simulink model "fft_overlap_tomori"  (R2023b)
settings: Solver=VariableStepAuto  StartTime=0.0  StopTime=inf  RelTol=1e-3
InitFcn:
  | fftparrallelout
  | load('dataram.mat')
  | s= fi(exp(-1j*2*pi.*(0:63)/64),1,16,15);
  | fixed_point = fixdt(1,27,20);
  | fixed_pointu = fixdt(0,29,20);
  | fixed = fixdt(1,22,15);
  | const = fixdt(1,18,17);
  | addConst = fixdt(1,18,16);
  | f =10.4e6;
  | f1=45e6;
  | alpha1 =5;
  | beta1 = 0.00001 ;
  | beta2 = 0.99999 ;
  | beta3 = 23;
undefined symbols (not defined in the file or in its folder): j
libraries: dspxfrm3 x11, commrflib2 x4
(part 3 of 10)

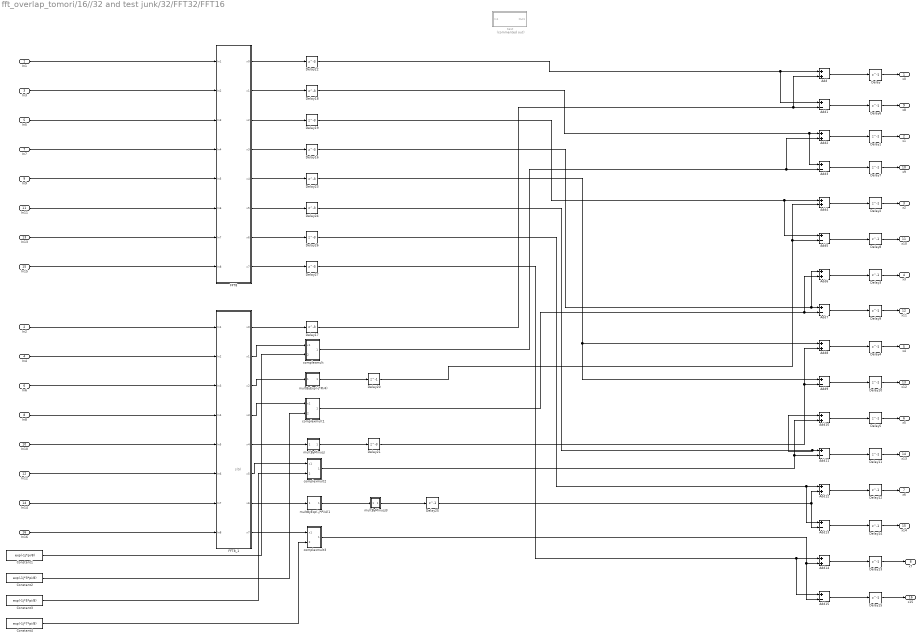
== system fft_overlap_tomori/16//32 and test junk/32/FFT32/FFT16 ==
  note: s(5)
  In1 : Inport
  In2 : Inport  Port=2
  In3 : Inport  Port=3
  In4 : Inport  Port=4
  In5 : Inport  Port=5
  In6 : Inport  Port=6
  In7 : Inport  Port=7
  In8 : Inport  Port=8
  In9 : Inport  Port=9
  In10 : Inport  Port=10
  In11 : Inport  Port=11
  In12 : Inport  Port=12
  In13 : Inport  Port=13
  In14 : Inport  Port=14
  In15 : Inport  Port=15
  In16 : Inport  Port=16
  Add{,2,4,6,8,10,12,14} (8 alike) : Sum  OutDataTypeStr=fixed
  Add{1,3,5,7,9,11,13,15} (8 alike) : Sum  Inputs=+-  OutDataTypeStr=fixed
  Constant1 : Constant  Value=exp(-1j*pi/8)  OutDataTypeStr=fixed  SampleTime=-1
  Constant2 : Constant  Value=exp(-1j*3*pi/8)  OutDataTypeStr=fixed  SampleTime=-1
  Constant3 : Constant  Value=exp(-1j*5*pi/8)  OutDataTypeStr=fixed  SampleTime=-1
  Constant4 : Constant  Value=exp(-1j*7*pi/8)  OutDataTypeStr=fixed  SampleTime=-1
  Delay{,1..15,20,25} (18 alike) : Delay  DelayLength=1
  Delay{16..19,21..24,26..27} (10 alike) : Delay  DelayLength=3
  FFT8 : Subsystem
  FFT8_1 : Subsystem
  complexmult : Subsystem
  complexmult1 : Subsystem
  complexmult2 : Subsystem
  complexmult3 : Subsystem
  multByExp(-j*Pi/4) : Subsystem
  multByExp(-j*Pi/4)1 : Subsystem
  multByMinusJ : Subsystem
  multByMinusJ3 : Subsystem
  test : Subsystem  Commented=on
  x0 : Outport
  x1 : Outport  Port=2
  x2 : Outport  Port=3
  x3 : Outport  Port=4
  x4 : Outport  Port=5
  x5 : Outport  Port=6
  x6 : Outport  Port=7
  x7 : Outport  Port=8
  x8 : Outport  Port=9
  x9 : Outport  Port=10
  x10 : Outport  Port=11
  x11 : Outport  Port=12
  x12 : Outport  Port=13
  x13 : Outport  Port=14
  x14 : Outport  Port=15
  x15 : Outport  Port=16
  wires:
  FFT8_1/1(x0) -> Delay17/1
  Add/1 -> Delay/1
  Add1/1 -> Delay6/1
  Constant1/1 -> complexmult/2(In3)
  FFT8_1/2(x1) -> complexmult/1(x1)
  FFT8/2(x1) -> Delay18/1
  Add2/1 -> Delay1/1
  complexmult/1(Out1) -> Add2/2, Add3/2
  Add3/1 -> Delay7/1
  FFT8_1/3(x2) -> multByExp(-j*Pi/4)/1(In1)
  FFT8/3(x2) -> Delay19/1
  Add4/1 -> Delay2/1
  Add5/1 -> Delay8/1
  multByExp(-j*Pi/4)/1(Out1) -> Delay20/1
  Constant2/1 -> complexmult1/2(In3)
  FFT8_1/4(x3) -> complexmult1/1(x1)
  FFT8/4(x3) -> Delay16/1
  complexmult1/1(Out1) -> Add6/2, Add7/2
  Add6/1 -> Delay3/1
  Add7/1 -> Delay9/1
  FFT8/5(x4) -> Delay23/1
  multByMinusJ/1(Out1) -> Delay21/1
  Add8/1 -> Delay4/1
  Add9/1 -> Delay10/1
  complexmult2/1(Out1) -> Add11/2, Add10/2
  FFT8/6(x5) -> Delay24/1
  Add10/1 -> Delay5/1
  Add11/1 -> Delay11/1
  Delay/1 -> x0/1
  Delay1/1 -> x1/1
  Delay2/1 -> x2/1
  Delay3/1 -> x3/1
  Delay4/1 -> x4/1
  Delay5/1 -> x5/1
  Delay6/1 -> x8/1
  Delay7/1 -> x9/1
  Delay8/1 -> x10/1
  Delay9/1 -> x11/1
  Delay10/1 -> x12/1
  Delay11/1 -> x13/1
  Delay12/1 -> x6/1
  Delay13/1 -> x7/1
  Delay14/1 -> x14/1
  Delay15/1 -> x15/1
  FFT8/1(x0) -> Delay22/1
  Delay17/1 -> Add/2, Add1/2
  Delay18/1 -> Add3/1, Add2/1
  Delay20/1 -> Add4/2, Add5/2
  Delay19/1 -> Add5/1, Add4/1
  Delay21/1 -> Add9/2, Add8/2
  FFT8_1/5(x4) -> multByMinusJ/1(x4)
  Delay22/1 -> Add1/1, Add/1
  Delay16/1 -> Add6/1, Add7/1
  Delay23/1 -> Add9/1, Add8/1
  Delay24/1 -> Add10/1, Add11/1
  FFT8_1/7(x6) -> multByExp(-j*Pi/4)1/1(In1)
  multByMinusJ3/1(Out1) -> Delay25/1
  FFT8/7(x6) -> Delay26/1
  Delay25/1 -> Add12/2, Add13/2
  Add12/1 -> Delay12/1
  Add13/1 -> Delay14/1
  Constant4/1 -> complexmult3/2(In3)
  FFT8_1/8(x7) -> complexmult3/1(x1)
  complexmult3/1(Out1) -> Add15/2, Add14/2
  FFT8/8(x7) -> Delay27/1
  Add14/1 -> Delay13/1
  Add15/1 -> Delay15/1
  Delay26/1 -> Add13/1, Add12/1
  Delay27/1 -> Add15/1, Add14/1
  FFT8_1/6(x5) -> complexmult2/1(x1)
  Constant3/1 -> complexmult2/2(In3)
  multByExp(-j*Pi/4)1/1(Out1) -> multByMinusJ3/1(In1)
  In1/1 -> FFT8/1(In1)
  In3/1 -> FFT8/2(In2)
  In5/1 -> FFT8/3(In3)
  In7/1 -> FFT8/4(In4)
  In9/1 -> FFT8/5(In5)
  In11/1 -> FFT8/6(In6)
  In13/1 -> FFT8/7(In7)
  In15/1 -> FFT8/8(In8)
  In2/1 -> FFT8_1/1(In1)
  In4/1 -> FFT8_1/2(In2)
  In6/1 -> FFT8_1/3(In3)
  In8/1 -> FFT8_1/4(In4)
  In10/1 -> FFT8_1/5(In5)
  In12/1 -> FFT8_1/6(In6)
  In14/1 -> FFT8_1/7(In7)
  In16/1 -> FFT8_1/8(In8)

== system fft_overlap_tomori/16//32 and test junk/32/FFT32/FFT16_1 ==
  note: s(5)
  In1 : Inport
  In2 : Inport  Port=2
  In3 : Inport  Port=3
  In4 : Inport  Port=4
  In5 : Inport  Port=5
  In6 : Inport  Port=6
  In7 : Inport  Port=7
  In8 : Inport  Port=8
  In9 : Inport  Port=9
  In10 : Inport  Port=10
  In11 : Inport  Port=11
  In12 : Inport  Port=12
  In13 : Inport  Port=13
  In14 : Inport  Port=14
  In15 : Inport  Port=15
  In16 : Inport  Port=16
  Add{,2,4,6,8,10,12,14} (8 alike) : Sum  OutDataTypeStr=fixed
  Add{1,3,5,7,9,11,13,15} (8 alike) : Sum  Inputs=+-  OutDataTypeStr=fixed
  Constant1 : Constant  Value=exp(-1j*pi/8)  OutDataTypeStr=fixed  SampleTime=-1
  Constant2 : Constant  Value=exp(-1j*3*pi/8)  OutDataTypeStr=fixed  SampleTime=-1
  Constant3 : Constant  Value=exp(-1j*5*pi/8)  OutDataTypeStr=fixed  SampleTime=-1
  Constant4 : Constant  Value=exp(-1j*7*pi/8)  OutDataTypeStr=fixed  SampleTime=-1
  Delay{,1..15,20,25} (18 alike) : Delay  DelayLength=1
  Delay{16..19,21..24,26..27} (10 alike) : Delay  DelayLength=3
  FFT8 : Subsystem
  FFT8_1 : Subsystem
  complexmult : Subsystem
  complexmult1 : Subsystem
  complexmult2 : Subsystem
  complexmult3 : Subsystem
  multByExp(-j*Pi/4) : Subsystem
  multByExp(-j*Pi/4)1 : Subsystem
  multByMinusJ : Subsystem
  multByMinusJ3 : Subsystem
  test : Subsystem  Commented=on
  x0 : Outport
  x1 : Outport  Port=2
  x2 : Outport  Port=3
  x3 : Outport  Port=4
  x4 : Outport  Port=5
  x5 : Outport  Port=6
  x6 : Outport  Port=7
  x7 : Outport  Port=8
  x8 : Outport  Port=9
  x9 : Outport  Port=10
  x10 : Outport  Port=11
  x11 : Outport  Port=12
  x12 : Outport  Port=13
  x13 : Outport  Port=14
  x14 : Outport  Port=15
  x15 : Outport  Port=16
  wires:
  In16/1 -> FFT8_1/8(In8)
  In14/1 -> FFT8_1/7(In7)
  In12/1 -> FFT8_1/6(In6)
  In10/1 -> FFT8_1/5(In5)
  In8/1 -> FFT8_1/4(In4)
  In6/1 -> FFT8_1/3(In3)
  In4/1 -> FFT8_1/2(In2)
  In2/1 -> FFT8_1/1(In1)
  In15/1 -> FFT8/8(In8)
  In13/1 -> FFT8/7(In7)
  In11/1 -> FFT8/6(In6)
  In9/1 -> FFT8/5(In5)
  In7/1 -> FFT8/4(In4)
  In5/1 -> FFT8/3(In3)
  In3/1 -> FFT8/2(In2)
  In1/1 -> FFT8/1(In1)
  multByExp(-j*Pi/4)1/1(Out1) -> multByMinusJ3/1(In1)
  Constant3/1 -> complexmult2/2(In3)
  FFT8_1/6(x5) -> complexmult2/1(x1)
  Delay27/1 -> Add14/1, Add15/1
  Delay26/1 -> Add12/1, Add13/1
  Add15/1 -> Delay15/1
  Add14/1 -> Delay13/1
  FFT8/8(x7) -> Delay27/1
  complexmult3/1(Out1) -> Add14/2, Add15/2
  FFT8_1/8(x7) -> complexmult3/1(x1)
  Constant4/1 -> complexmult3/2(In3)
  Add13/1 -> Delay14/1
  Add12/1 -> Delay12/1
  Delay25/1 -> Add13/2, Add12/2
  FFT8/7(x6) -> Delay26/1
  multByMinusJ3/1(Out1) -> Delay25/1
  FFT8_1/7(x6) -> multByExp(-j*Pi/4)1/1(In1)
  Delay24/1 -> Add11/1, Add10/1
  Delay23/1 -> Add8/1, Add9/1
  Delay16/1 -> Add7/1, Add6/1
  Delay22/1 -> Add/1, Add1/1
  FFT8_1/5(x4) -> multByMinusJ/1(x4)
  Delay21/1 -> Add8/2, Add9/2
  Delay19/1 -> Add4/1, Add5/1
  Delay20/1 -> Add5/2, Add4/2
  Delay18/1 -> Add2/1, Add3/1
  Delay17/1 -> Add1/2, Add/2
  FFT8/1(x0) -> Delay22/1
  Delay15/1 -> x15/1
  Delay14/1 -> x14/1
  Delay13/1 -> x7/1
  Delay12/1 -> x6/1
  Delay11/1 -> x13/1
  Delay10/1 -> x12/1
  Delay9/1 -> x11/1
  Delay8/1 -> x10/1
  Delay7/1 -> x9/1
  Delay6/1 -> x8/1
  Delay5/1 -> x5/1
  Delay4/1 -> x4/1
  Delay3/1 -> x3/1
  Delay2/1 -> x2/1
  Delay1/1 -> x1/1
  Delay/1 -> x0/1
  Add11/1 -> Delay11/1
  Add10/1 -> Delay5/1
  FFT8/6(x5) -> Delay24/1
  complexmult2/1(Out1) -> Add10/2, Add11/2
  Add9/1 -> Delay10/1
  Add8/1 -> Delay4/1
  multByMinusJ/1(Out1) -> Delay21/1
  FFT8/5(x4) -> Delay23/1
  Add7/1 -> Delay9/1
  Add6/1 -> Delay3/1
  complexmult1/1(Out1) -> Add7/2, Add6/2
  FFT8/4(x3) -> Delay16/1
  FFT8_1/4(x3) -> complexmult1/1(x1)
  Constant2/1 -> complexmult1/2(In3)
  multByExp(-j*Pi/4)/1(Out1) -> Delay20/1
  Add5/1 -> Delay8/1
  Add4/1 -> Delay2/1
  FFT8/3(x2) -> Delay19/1
  FFT8_1/3(x2) -> multByExp(-j*Pi/4)/1(In1)
  Add3/1 -> Delay7/1
  complexmult/1(Out1) -> Add3/2, Add2/2
  Add2/1 -> Delay1/1
  FFT8/2(x1) -> Delay18/1
  FFT8_1/2(x1) -> complexmult/1(x1)
  Constant1/1 -> complexmult/2(In3)
  Add1/1 -> Delay6/1
  Add/1 -> Delay/1
  FFT8_1/1(x0) -> Delay17/1

== system fft_overlap_tomori/16//32 and test junk/32/FFT32/complexmult ==
  x1 : Inport
  In3 : Inport  Port=2
  Add1 : Sum  OutDataTypeStr=fixed  RndMeth=Round
  Add20 : Sum  OutDataTypeStr=fixed  RndMeth=Round
  Add3 : Sum  Inputs=+--  OutDataTypeStr=fixed  AccumDataTypeStr=fixed  RndMeth=Round
  Add4 : Sum  Inputs=+-  OutDataTypeStr=fixed  AccumDataTypeStr=fixed  RndMeth=Round
  Complex to Real-Imag : ComplexToRealImag
  Complex to Real-Imag1 : ComplexToRealImag
  Constant : Constant  Commented=on  Value=1+j  OutDataTypeStr=fixdt(1,22, 15)  SampleTime=2e-8
  Constant1 : Constant  Commented=on  Value=1-j  OutDataTypeStr=fixdt(1,22, 15)  SampleTime=2e-8
  Delay : Delay  DelayLength=3
  Delay1 : Delay  DelayLength=3
  Delay2 : Delay  DelayLength=3
  Display : Display  Commented=on
  Product : Product  OutDataTypeStr=fixed  RndMeth=Round
  Product1 : Product  OutDataTypeStr=fixed  RndMeth=Round
  Product2 : Product  OutDataTypeStr=fixed  RndMeth=Round
  Real-Imag to Complex : RealImagToComplex
  Out1 : Outport
  wires:
  Real-Imag to Complex/1 -> Out1/1
  In3/1 -> Complex to Real-Imag1/1
  x1/1 -> Complex to Real-Imag/1
  Product/1 -> Delay/1
  Product1/1 -> Delay1/1
  Product2/1 -> Delay2/1
  Delay/1 -> Add3/1
  Delay1/1 -> Add4/1, Add3/2
  Delay2/1 -> Add3/3, Add4/2
  Add4/1 -> Real-Imag to Complex/1
  Add3/1 -> Real-Imag to Complex/2
  Add20/1 -> Product/1
  Add1/1 -> Product/2
  Complex to Real-Imag/1 -> Product1/1, Add20/1
  Complex to Real-Imag1/1 -> Product1/2, Add1/1
  Complex to Real-Imag/2 -> Product2/1, Add20/2
  Complex to Real-Imag1/2 -> Product2/2, Add1/2

== system fft_overlap_tomori/16//32 and test junk/32/FFT32/complexmult1 ==
  x1 : Inport
  In3 : Inport  Port=2
  Add1 : Sum  OutDataTypeStr=fixed  RndMeth=Round
  Add20 : Sum  OutDataTypeStr=fixed  RndMeth=Round
  Add3 : Sum  Inputs=+--  OutDataTypeStr=fixed  AccumDataTypeStr=fixed  RndMeth=Round
  Add4 : Sum  Inputs=+-  OutDataTypeStr=fixed  AccumDataTypeStr=fixed  RndMeth=Round
  Complex to Real-Imag : ComplexToRealImag
  Complex to Real-Imag1 : ComplexToRealImag
  Constant : Constant  Commented=on  Value=1+j  OutDataTypeStr=fixdt(1,22, 15)  SampleTime=2e-8
  Constant1 : Constant  Commented=on  Value=1-j  OutDataTypeStr=fixdt(1,22, 15)  SampleTime=2e-8
  Delay : Delay  DelayLength=3
  Delay1 : Delay  DelayLength=3
  Delay2 : Delay  DelayLength=3
  Display : Display  Commented=on
  Product : Product  OutDataTypeStr=fixed  RndMeth=Round
  Product1 : Product  OutDataTypeStr=fixed  RndMeth=Round
  Product2 : Product  OutDataTypeStr=fixed  RndMeth=Round
  Real-Imag to Complex : RealImagToComplex
  Out1 : Outport
  wires:
  Complex to Real-Imag1/2 -> Add1/2, Product2/2
  Complex to Real-Imag/2 -> Add20/2, Product2/1
  Complex to Real-Imag1/1 -> Add1/1, Product1/2
  Complex to Real-Imag/1 -> Add20/1, Product1/1
  Add1/1 -> Product/2
  Add20/1 -> Product/1
  Add3/1 -> Real-Imag to Complex/2
  Add4/1 -> Real-Imag to Complex/1
  Delay2/1 -> Add4/2, Add3/3
  Delay1/1 -> Add3/2, Add4/1
  Delay/1 -> Add3/1
  Product2/1 -> Delay2/1
  Product1/1 -> Delay1/1
  Product/1 -> Delay/1
  x1/1 -> Complex to Real-Imag/1
  In3/1 -> Complex to Real-Imag1/1
  Real-Imag to Complex/1 -> Out1/1

== system fft_overlap_tomori/16//32 and test junk/32/FFT32/complexmult10 ==
  x1 : Inport
  In3 : Inport  Port=2
  Add1 : Sum  OutDataTypeStr=fixed  RndMeth=Round
  Add20 : Sum  OutDataTypeStr=fixed  RndMeth=Round
  Add3 : Sum  Inputs=+--  OutDataTypeStr=fixed  AccumDataTypeStr=fixed  RndMeth=Round
  Add4 : Sum  Inputs=+-  OutDataTypeStr=fixed  AccumDataTypeStr=fixed  RndMeth=Round
  Complex to Real-Imag : ComplexToRealImag
  Complex to Real-Imag1 : ComplexToRealImag
  Constant : Constant  Commented=on  Value=1+j  OutDataTypeStr=fixdt(1,22, 15)  SampleTime=2e-8
  Constant1 : Constant  Commented=on  Value=1-j  OutDataTypeStr=fixdt(1,22, 15)  SampleTime=2e-8
  Delay : Delay  DelayLength=3
  Delay1 : Delay  DelayLength=3
  Delay2 : Delay  DelayLength=3
  Display : Display  Commented=on
  Product : Product  OutDataTypeStr=fixed  RndMeth=Round
  Product1 : Product  OutDataTypeStr=fixed  RndMeth=Round
  Product2 : Product  OutDataTypeStr=fixed  RndMeth=Round
  Real-Imag to Complex : RealImagToComplex
  Out1 : Outport
  wires:
  Real-Imag to Complex/1 -> Out1/1
  In3/1 -> Complex to Real-Imag1/1
  x1/1 -> Complex to Real-Imag/1
  Product/1 -> Delay/1
  Product1/1 -> Delay1/1
  Product2/1 -> Delay2/1
  Delay/1 -> Add3/1
  Delay1/1 -> Add4/1, Add3/2
  Delay2/1 -> Add3/3, Add4/2
  Add4/1 -> Real-Imag to Complex/1
  Add3/1 -> Real-Imag to Complex/2
  Add20/1 -> Product/1
  Add1/1 -> Product/2
  Complex to Real-Imag/1 -> Product1/1, Add20/1
  Complex to Real-Imag1/1 -> Product1/2, Add1/1
  Complex to Real-Imag/2 -> Product2/1, Add20/2
  Complex to Real-Imag1/2 -> Product2/2, Add1/2

== system fft_overlap_tomori/16//32 and test junk/32/FFT32/complexmult11 ==
  x1 : Inport
  In3 : Inport  Port=2
  Add1 : Sum  OutDataTypeStr=fixed  RndMeth=Round
  Add20 : Sum  OutDataTypeStr=fixed  RndMeth=Round
  Add3 : Sum  Inputs=+--  OutDataTypeStr=fixed  AccumDataTypeStr=fixed  RndMeth=Round
  Add4 : Sum  Inputs=+-  OutDataTypeStr=fixed  AccumDataTypeStr=fixed  RndMeth=Round
  Complex to Real-Imag : ComplexToRealImag
  Complex to Real-Imag1 : ComplexToRealImag
  Constant : Constant  Commented=on  Value=1+j  OutDataTypeStr=fixdt(1,22, 15)  SampleTime=2e-8
  Constant1 : Constant  Commented=on  Value=1-j  OutDataTypeStr=fixdt(1,22, 15)  SampleTime=2e-8
  Delay : Delay  DelayLength=3
  Delay1 : Delay  DelayLength=3
  Delay2 : Delay  DelayLength=3
  Display : Display  Commented=on
  Product : Product  OutDataTypeStr=fixed  RndMeth=Round
  Product1 : Product  OutDataTypeStr=fixed  RndMeth=Round
  Product2 : Product  OutDataTypeStr=fixed  RndMeth=Round
  Real-Imag to Complex : RealImagToComplex
  Out1 : Outport
  wires:
  Complex to Real-Imag1/2 -> Add1/2, Product2/2
  Complex to Real-Imag/2 -> Add20/2, Product2/1
  Complex to Real-Imag1/1 -> Add1/1, Product1/2
  Complex to Real-Imag/1 -> Add20/1, Product1/1
  Add1/1 -> Product/2
  Add20/1 -> Product/1
  Add3/1 -> Real-Imag to Complex/2
  Add4/1 -> Real-Imag to Complex/1
  Delay2/1 -> Add4/2, Add3/3
  Delay1/1 -> Add3/2, Add4/1
  Delay/1 -> Add3/1
  Product2/1 -> Delay2/1
  Product1/1 -> Delay1/1
  Product/1 -> Delay/1
  x1/1 -> Complex to Real-Imag/1
  In3/1 -> Complex to Real-Imag1/1
  Real-Imag to Complex/1 -> Out1/1

== system fft_overlap_tomori/16//32 and test junk/32/FFT32/complexmult2 ==
  x1 : Inport
  In3 : Inport  Port=2
  Add1 : Sum  OutDataTypeStr=fixed  RndMeth=Round
  Add20 : Sum  OutDataTypeStr=fixed  RndMeth=Round
  Add3 : Sum  Inputs=+--  OutDataTypeStr=fixed  AccumDataTypeStr=fixed  RndMeth=Round
  Add4 : Sum  Inputs=+-  OutDataTypeStr=fixed  AccumDataTypeStr=fixed  RndMeth=Round
  Complex to Real-Imag : ComplexToRealImag
  Complex to Real-Imag1 : ComplexToRealImag
  Constant : Constant  Commented=on  Value=1+j  OutDataTypeStr=fixdt(1,22, 15)  SampleTime=2e-8
  Constant1 : Constant  Commented=on  Value=1-j  OutDataTypeStr=fixdt(1,22, 15)  SampleTime=2e-8
  Delay : Delay  DelayLength=3
  Delay1 : Delay  DelayLength=3
  Delay2 : Delay  DelayLength=3
  Display : Display  Commented=on
  Product : Product  OutDataTypeStr=fixed  RndMeth=Round
  Product1 : Product  OutDataTypeStr=fixed  RndMeth=Round
  Product2 : Product  OutDataTypeStr=fixed  RndMeth=Round
  Real-Imag to Complex : RealImagToComplex
  Out1 : Outport
  wires:
  Real-Imag to Complex/1 -> Out1/1
  In3/1 -> Complex to Real-Imag1/1
  x1/1 -> Complex to Real-Imag/1
  Product/1 -> Delay/1
  Product1/1 -> Delay1/1
  Product2/1 -> Delay2/1
  Delay/1 -> Add3/1
  Delay1/1 -> Add4/1, Add3/2
  Delay2/1 -> Add3/3, Add4/2
  Add4/1 -> Real-Imag to Complex/1
  Add3/1 -> Real-Imag to Complex/2
  Add20/1 -> Product/1
  Add1/1 -> Product/2
  Complex to Real-Imag/1 -> Product1/1, Add20/1
  Complex to Real-Imag1/1 -> Product1/2, Add1/1
  Complex to Real-Imag/2 -> Product2/1, Add20/2
  Complex to Real-Imag1/2 -> Product2/2, Add1/2

== system fft_overlap_tomori/16//32 and test junk/32/FFT32/complexmult3 ==
  x1 : Inport
  In3 : Inport  Port=2
  Add1 : Sum  OutDataTypeStr=fixed  RndMeth=Round
  Add20 : Sum  OutDataTypeStr=fixed  RndMeth=Round
  Add3 : Sum  Inputs=+--  OutDataTypeStr=fixed  AccumDataTypeStr=fixed  RndMeth=Round
  Add4 : Sum  Inputs=+-  OutDataTypeStr=fixed  AccumDataTypeStr=fixed  RndMeth=Round
  Complex to Real-Imag : ComplexToRealImag
  Complex to Real-Imag1 : ComplexToRealImag
  Constant : Constant  Commented=on  Value=1+j  OutDataTypeStr=fixdt(1,22, 15)  SampleTime=2e-8
  Constant1 : Constant  Commented=on  Value=1-j  OutDataTypeStr=fixdt(1,22, 15)  SampleTime=2e-8
  Delay : Delay  DelayLength=3
  Delay1 : Delay  DelayLength=3
  Delay2 : Delay  DelayLength=3
  Display : Display  Commented=on
  Product : Product  OutDataTypeStr=fixed  RndMeth=Round
  Product1 : Product  OutDataTypeStr=fixed  RndMeth=Round
  Product2 : Product  OutDataTypeStr=fixed  RndMeth=Round
  Real-Imag to Complex : RealImagToComplex
  Out1 : Outport
  wires:
  Complex to Real-Imag1/2 -> Add1/2, Product2/2
  Complex to Real-Imag/2 -> Add20/2, Product2/1
  Complex to Real-Imag1/1 -> Add1/1, Product1/2
  Complex to Real-Imag/1 -> Add20/1, Product1/1
  Add1/1 -> Product/2
  Add20/1 -> Product/1
  Add3/1 -> Real-Imag to Complex/2
  Add4/1 -> Real-Imag to Complex/1
  Delay2/1 -> Add4/2, Add3/3
  Delay1/1 -> Add3/2, Add4/1
  Delay/1 -> Add3/1
  Product2/1 -> Delay2/1
  Product1/1 -> Delay1/1
  Product/1 -> Delay/1
  x1/1 -> Complex to Real-Imag/1
  In3/1 -> Complex to Real-Imag1/1
  Real-Imag to Complex/1 -> Out1/1

== system fft_overlap_tomori/16//32 and test junk/32/FFT32/complexmult4 ==
  x1 : Inport
  In3 : Inport  Port=2
  Add1 : Sum  OutDataTypeStr=fixed  RndMeth=Round
  Add20 : Sum  OutDataTypeStr=fixed  RndMeth=Round
  Add3 : Sum  Inputs=+--  OutDataTypeStr=fixed  AccumDataTypeStr=fixed  RndMeth=Round
  Add4 : Sum  Inputs=+-  OutDataTypeStr=fixed  AccumDataTypeStr=fixed  RndMeth=Round
  Complex to Real-Imag : ComplexToRealImag
  Complex to Real-Imag1 : ComplexToRealImag
  Constant : Constant  Commented=on  Value=1+j  OutDataTypeStr=fixdt(1,22, 15)  SampleTime=2e-8
  Constant1 : Constant  Commented=on  Value=1-j  OutDataTypeStr=fixdt(1,22, 15)  SampleTime=2e-8
  Delay : Delay  DelayLength=3
  Delay1 : Delay  DelayLength=3
  Delay2 : Delay  DelayLength=3
  Display : Display  Commented=on
  Product : Product  OutDataTypeStr=fixed  RndMeth=Round
  Product1 : Product  OutDataTypeStr=fixed  RndMeth=Round
  Product2 : Product  OutDataTypeStr=fixed  RndMeth=Round
  Real-Imag to Complex : RealImagToComplex
  Out1 : Outport
  wires:
  Real-Imag to Complex/1 -> Out1/1
  In3/1 -> Complex to Real-Imag1/1
  x1/1 -> Complex to Real-Imag/1
  Product/1 -> Delay/1
  Product1/1 -> Delay1/1
  Product2/1 -> Delay2/1
  Delay/1 -> Add3/1
  Delay1/1 -> Add4/1, Add3/2
  Delay2/1 -> Add3/3, Add4/2
  Add4/1 -> Real-Imag to Complex/1
  Add3/1 -> Real-Imag to Complex/2
  Add20/1 -> Product/1
  Add1/1 -> Product/2
  Complex to Real-Imag/1 -> Product1/1, Add20/1
  Complex to Real-Imag1/1 -> Product1/2, Add1/1
  Complex to Real-Imag/2 -> Product2/1, Add20/2
  Complex to Real-Imag1/2 -> Product2/2, Add1/2

== system fft_overlap_tomori/16//32 and test junk/32/FFT32/complexmult5 ==
  x1 : Inport
  In3 : Inport  Port=2
  Add1 : Sum  OutDataTypeStr=fixed  RndMeth=Round
  Add20 : Sum  OutDataTypeStr=fixed  RndMeth=Round
  Add3 : Sum  Inputs=+--  OutDataTypeStr=fixed  AccumDataTypeStr=fixed  RndMeth=Round
  Add4 : Sum  Inputs=+-  OutDataTypeStr=fixed  AccumDataTypeStr=fixed  RndMeth=Round
  Complex to Real-Imag : ComplexToRealImag
  Complex to Real-Imag1 : ComplexToRealImag
  Constant : Constant  Commented=on  Value=1+j  OutDataTypeStr=fixdt(1,22, 15)  SampleTime=2e-8
  Constant1 : Constant  Commented=on  Value=1-j  OutDataTypeStr=fixdt(1,22, 15)  SampleTime=2e-8
  Delay : Delay  DelayLength=3
  Delay1 : Delay  DelayLength=3
  Delay2 : Delay  DelayLength=3
  Display : Display  Commented=on
  Product : Product  OutDataTypeStr=fixed  RndMeth=Round
  Product1 : Product  OutDataTypeStr=fixed  RndMeth=Round
  Product2 : Product  OutDataTypeStr=fixed  RndMeth=Round
  Real-Imag to Complex : RealImagToComplex
  Out1 : Outport
  wires:
  Complex to Real-Imag1/2 -> Add1/2, Product2/2
  Complex to Real-Imag/2 -> Add20/2, Product2/1
  Complex to Real-Imag1/1 -> Add1/1, Product1/2
  Complex to Real-Imag/1 -> Add20/1, Product1/1
  Add1/1 -> Product/2
  Add20/1 -> Product/1
  Add3/1 -> Real-Imag to Complex/2
  Add4/1 -> Real-Imag to Complex/1
  Delay2/1 -> Add4/2, Add3/3
  Delay1/1 -> Add3/2, Add4/1
  Delay/1 -> Add3/1
  Product2/1 -> Delay2/1
  Product1/1 -> Delay1/1
  Product/1 -> Delay/1
  x1/1 -> Complex to Real-Imag/1
  In3/1 -> Complex to Real-Imag1/1
  Real-Imag to Complex/1 -> Out1/1

== system fft_overlap_tomori/16//32 and test junk/32/FFT32/complexmult6 ==
  x1 : Inport
  In3 : Inport  Port=2
  Add1 : Sum  OutDataTypeStr=fixed  RndMeth=Round
  Add20 : Sum  OutDataTypeStr=fixed  RndMeth=Round
  Add3 : Sum  Inputs=+--  OutDataTypeStr=fixed  AccumDataTypeStr=fixed  RndMeth=Round
  Add4 : Sum  Inputs=+-  OutDataTypeStr=fixed  AccumDataTypeStr=fixed  RndMeth=Round
  Complex to Real-Imag : ComplexToRealImag
  Complex to Real-Imag1 : ComplexToRealImag
  Constant : Constant  Commented=on  Value=1+j  OutDataTypeStr=fixdt(1,22, 15)  SampleTime=2e-8
  Constant1 : Constant  Commented=on  Value=1-j  OutDataTypeStr=fixdt(1,22, 15)  SampleTime=2e-8
  Delay : Delay  DelayLength=3
  Delay1 : Delay  DelayLength=3
  Delay2 : Delay  DelayLength=3
  Display : Display  Commented=on
  Product : Product  OutDataTypeStr=fixed  RndMeth=Round
  Product1 : Product  OutDataTypeStr=fixed  RndMeth=Round
  Product2 : Product  OutDataTypeStr=fixed  RndMeth=Round
  Real-Imag to Complex : RealImagToComplex
  Out1 : Outport
  wires:
  Real-Imag to Complex/1 -> Out1/1
  In3/1 -> Complex to Real-Imag1/1
  x1/1 -> Complex to Real-Imag/1
  Product/1 -> Delay/1
  Product1/1 -> Delay1/1
  Product2/1 -> Delay2/1
  Delay/1 -> Add3/1
  Delay1/1 -> Add4/1, Add3/2
  Delay2/1 -> Add3/3, Add4/2
  Add4/1 -> Real-Imag to Complex/1
  Add3/1 -> Real-Imag to Complex/2
  Add20/1 -> Product/1
  Add1/1 -> Product/2
  Complex to Real-Imag/1 -> Product1/1, Add20/1
  Complex to Real-Imag1/1 -> Product1/2, Add1/1
  Complex to Real-Imag/2 -> Product2/1, Add20/2
  Complex to Real-Imag1/2 -> Product2/2, Add1/2

== system fft_overlap_tomori/16//32 and test junk/32/FFT32/complexmult7 ==
  x1 : Inport
  In3 : Inport  Port=2
  Add1 : Sum  OutDataTypeStr=fixed  RndMeth=Round
  Add20 : Sum  OutDataTypeStr=fixed  RndMeth=Round
  Add3 : Sum  Inputs=+--  OutDataTypeStr=fixed  AccumDataTypeStr=fixed  RndMeth=Round
  Add4 : Sum  Inputs=+-  OutDataTypeStr=fixed  AccumDataTypeStr=fixed  RndMeth=Round
  Complex to Real-Imag : ComplexToRealImag
  Complex to Real-Imag1 : ComplexToRealImag
  Constant : Constant  Commented=on  Value=1+j  OutDataTypeStr=fixdt(1,22, 15)  SampleTime=2e-8
  Constant1 : Constant  Commented=on  Value=1-j  OutDataTypeStr=fixdt(1,22, 15)  SampleTime=2e-8
  Delay : Delay  DelayLength=3
  Delay1 : Delay  DelayLength=3
  Delay2 : Delay  DelayLength=3
  Display : Display  Commented=on
  Product : Product  OutDataTypeStr=fixed  RndMeth=Round
  Product1 : Product  OutDataTypeStr=fixed  RndMeth=Round
  Product2 : Product  OutDataTypeStr=fixed  RndMeth=Round
  Real-Imag to Complex : RealImagToComplex
  Out1 : Outport
  wires:
  Complex to Real-Imag1/2 -> Add1/2, Product2/2
  Complex to Real-Imag/2 -> Add20/2, Product2/1
  Complex to Real-Imag1/1 -> Add1/1, Product1/2
  Complex to Real-Imag/1 -> Add20/1, Product1/1
  Add1/1 -> Product/2
  Add20/1 -> Product/1
  Add3/1 -> Real-Imag to Complex/2
  Add4/1 -> Real-Imag to Complex/1
  Delay2/1 -> Add4/2, Add3/3
  Delay1/1 -> Add3/2, Add4/1
  Delay/1 -> Add3/1
  Product2/1 -> Delay2/1
  Product1/1 -> Delay1/1
  Product/1 -> Delay/1
  x1/1 -> Complex to Real-Imag/1
  In3/1 -> Complex to Real-Imag1/1
  Real-Imag to Complex/1 -> Out1/1

== system fft_overlap_tomori/16//32 and test junk/32/FFT32/complexmult8 ==
  x1 : Inport
  In3 : Inport  Port=2
  Add1 : Sum  OutDataTypeStr=fixed  RndMeth=Round
  Add20 : Sum  OutDataTypeStr=fixed  RndMeth=Round
  Add3 : Sum  Inputs=+--  OutDataTypeStr=fixed  AccumDataTypeStr=fixed  RndMeth=Round
  Add4 : Sum  Inputs=+-  OutDataTypeStr=fixed  AccumDataTypeStr=fixed  RndMeth=Round
  Complex to Real-Imag : ComplexToRealImag
  Complex to Real-Imag1 : ComplexToRealImag
  Constant : Constant  Commented=on  Value=1+j  OutDataTypeStr=fixdt(1,22, 15)  SampleTime=2e-8
  Constant1 : Constant  Commented=on  Value=1-j  OutDataTypeStr=fixdt(1,22, 15)  SampleTime=2e-8
  Delay : Delay  DelayLength=3
  Delay1 : Delay  DelayLength=3
  Delay2 : Delay  DelayLength=3
  Display : Display  Commented=on
  Product : Product  OutDataTypeStr=fixed  RndMeth=Round
  Product1 : Product  OutDataTypeStr=fixed  RndMeth=Round
  Product2 : Product  OutDataTypeStr=fixed  RndMeth=Round
  Real-Imag to Complex : RealImagToComplex
  Out1 : Outport
  wires:
  Real-Imag to Complex/1 -> Out1/1
  In3/1 -> Complex to Real-Imag1/1
  x1/1 -> Complex to Real-Imag/1
  Product/1 -> Delay/1
  Product1/1 -> Delay1/1
  Product2/1 -> Delay2/1
  Delay/1 -> Add3/1
  Delay1/1 -> Add4/1, Add3/2
  Delay2/1 -> Add3/3, Add4/2
  Add4/1 -> Real-Imag to Complex/1
  Add3/1 -> Real-Imag to Complex/2
  Add20/1 -> Product/1
  Add1/1 -> Product/2
  Complex to Real-Imag/1 -> Product1/1, Add20/1
  Complex to Real-Imag1/1 -> Product1/2, Add1/1
  Complex to Real-Imag/2 -> Product2/1, Add20/2
  Complex to Real-Imag1/2 -> Product2/2, Add1/2

== system fft_overlap_tomori/16//32 and test junk/32/FFT32/complexmult9 ==
  x1 : Inport
  In3 : Inport  Port=2
  Add1 : Sum  OutDataTypeStr=fixed  RndMeth=Round
  Add20 : Sum  OutDataTypeStr=fixed  RndMeth=Round
  Add3 : Sum  Inputs=+--  OutDataTypeStr=fixed  AccumDataTypeStr=fixed  RndMeth=Round
  Add4 : Sum  Inputs=+-  OutDataTypeStr=fixed  AccumDataTypeStr=fixed  RndMeth=Round
  Complex to Real-Imag : ComplexToRealImag
  Complex to Real-Imag1 : ComplexToRealImag
  Constant : Constant  Commented=on  Value=1+j  OutDataTypeStr=fixdt(1,22, 15)  SampleTime=2e-8
  Constant1 : Constant  Commented=on  Value=1-j  OutDataTypeStr=fixdt(1,22, 15)  SampleTime=2e-8
  Delay : Delay  DelayLength=3
  Delay1 : Delay  DelayLength=3
  Delay2 : Delay  DelayLength=3
  Display : Display  Commented=on
  Product : Product  OutDataTypeStr=fixed  RndMeth=Round
  Product1 : Product  OutDataTypeStr=fixed  RndMeth=Round
  Product2 : Product  OutDataTypeStr=fixed  RndMeth=Round
  Real-Imag to Complex : RealImagToComplex
  Out1 : Outport
  wires:
  Complex to Real-Imag1/2 -> Add1/2, Product2/2
  Complex to Real-Imag/2 -> Add20/2, Product2/1
  Complex to Real-Imag1/1 -> Add1/1, Product1/2
  Complex to Real-Imag/1 -> Add20/1, Product1/1
  Add1/1 -> Product/2
  Add20/1 -> Product/1
  Add3/1 -> Real-Imag to Complex/2
  Add4/1 -> Real-Imag to Complex/1
  Delay2/1 -> Add4/2, Add3/3
  Delay1/1 -> Add3/2, Add4/1
  Delay/1 -> Add3/1
  Product2/1 -> Delay2/1
  Product1/1 -> Delay1/1
  Product/1 -> Delay/1
  x1/1 -> Complex to Real-Imag/1
  In3/1 -> Complex to Real-Imag1/1
  Real-Imag to Complex/1 -> Out1/1

== system fft_overlap_tomori/16//32 and test junk/32/FFT32/multByExp(-j*Pi//4) ==
  x4 : Inport
  Add : Sum  OutDataTypeStr=fixed  RndMeth=Round
  Add1 : Sum  Inputs=+-  OutDataTypeStr=fixed  RndMeth=Round
  Complex to Real-Imag : ComplexToRealImag
  Delay24 : Delay
  Gain : Gain  Gain=sqrt(2)/2  ParamDataTypeStr=fixed  OutDataTypeStr=fixed  RndMeth=Round
  Real-Imag to Complex : RealImagToComplex
  Out1 : Outport
  wires:
  x4/1 -> Gain/1
  Real-Imag to Complex/1 -> Out1/1
  Delay24/1 -> Complex to Real-Imag/1
  Add1/1 -> Real-Imag to Complex/2
  Add/1 -> Real-Imag to Complex/1
  Complex to Real-Imag/2 -> Add/2, Add1/1
  Complex to Real-Imag/1 -> Add/1, Add1/2
  Gain/1 -> Delay24/1

== system fft_overlap_tomori/16//32 and test junk/32/FFT32/multByExp(-j*Pi//4)1 ==
  x4 : Inport
  Add : Sum  OutDataTypeStr=fixed  RndMeth=Round
  Add1 : Sum  Inputs=+-  OutDataTypeStr=fixed  RndMeth=Round
  Complex to Real-Imag : ComplexToRealImag
  Delay24 : Delay
  Gain : Gain  Gain=sqrt(2)/2  ParamDataTypeStr=fixed  OutDataTypeStr=fixed  RndMeth=Round
  Real-Imag to Complex : RealImagToComplex
  Out1 : Outport
  wires:
  x4/1 -> Gain/1
  Real-Imag to Complex/1 -> Out1/1
  Delay24/1 -> Complex to Real-Imag/1
  Add1/1 -> Real-Imag to Complex/2
  Add/1 -> Real-Imag to Complex/1
  Complex to Real-Imag/2 -> Add/2, Add1/1
  Complex to Real-Imag/1 -> Add/1, Add1/2
  Gain/1 -> Delay24/1

== system fft_overlap_tomori/16//32 and test junk/32/FFT32/multByMinusJ ==
  x4 : Inport
  Complex to Real-Imag : ComplexToRealImag
  Real-Imag to Complex : RealImagToComplex
  Unary Minus1 : UnaryMinus
  Out1 : Outport
  wires:
  Complex to Real-Imag/1 -> Unary Minus1/1
  Complex to Real-Imag/2 -> Real-Imag to Complex/1
  x4/1 -> Complex to Real-Imag/1
  Real-Imag to Complex/1 -> Out1/1
  Unary Minus1/1 -> Real-Imag to Complex/2

== system fft_overlap_tomori/16//32 and test junk/32/FFT32/multByMinusJ3 ==
  In1 : Inport
  Complex to Real-Imag : ComplexToRealImag
  Real-Imag to Complex : RealImagToComplex
  Unary Minus1 : UnaryMinus
  Out1 : Outport
  wires:
  Complex to Real-Imag/1 -> Unary Minus1/1
  Complex to Real-Imag/2 -> Real-Imag to Complex/1
  In1/1 -> Complex to Real-Imag/1
  Real-Imag to Complex/1 -> Out1/1
  Unary Minus1/1 -> Real-Imag to Complex/2

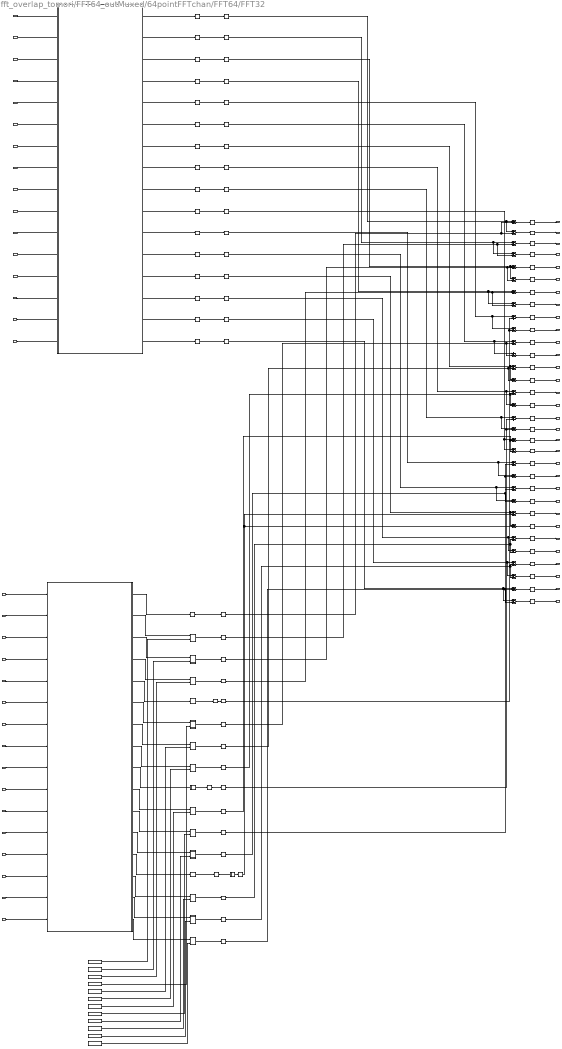
== system fft_overlap_tomori/FFT64_outMuxed/64pointFFTchan/FFT64/FFT32 ==
  In1 : Inport
  In2 : Inport  Port=2
  In3 : Inport  Port=3
  In4 : Inport  Port=4
  In5 : Inport  Port=5
  In6 : Inport  Port=6
  In7 : Inport  Port=7
  In8 : Inport  Port=8
  In9 : Inport  Port=9
  In10 : Inport  Port=10
  In11 : Inport  Port=11
  In12 : Inport  Port=12
  In13 : Inport  Port=13
  In14 : Inport  Port=14
  In15 : Inport  Port=15
  In17 : Inport  Port=16
  In19 : Inport  Port=17
  In16 : Inport  Port=18
  In18 : Inport  Port=19
  In20 : Inport  Port=20
  In21 : Inport  Port=21
  In22 : Inport  Port=22
  In23 : Inport  Port=23
  In24 : Inport  Port=24
  In25 : Inport  Port=25
  In26 : Inport  Port=26
  In27 : Inport  Port=27
  In28 : Inport  Port=28
  In29 : Inport  Port=29
  In30 : Inport  Port=30
  In31 : Inport  Port=31
  In32 : Inport  Port=32
  Add{,2,4,6,8,10,12,14,16,18,20,22,24,26,28,30} (16 alike) : Sum  OutDataTypeStr=fixed  RndMeth=Round
  Add{1,3,5,7,9,11,13,15,17,19,21,23,25,27,29,31} (16 alike) : Sum  Inputs=+-  OutDataTypeStr=fixed  RndMeth=Round
  Constant1 : Constant  Value=exp(-1j*pi/8)  OutDataTypeStr=const  SampleTime=-1
  Constant10 : Constant  Value=exp(-1j*pi*13/16)  OutDataTypeStr=const  SampleTime=-1
  Constant12 : Constant  Value=exp(-1j*7*pi/8)  OutDataTypeStr=const  SampleTime=-1
  Constant13 : Constant  Value=exp(-1j*pi*15/16)  OutDataTypeStr=const  SampleTime=-1
  Constant2 : Constant  Value=exp(-1j*pi/16)  OutDataTypeStr=const  SampleTime=-1
  Constant3 : Constant  Value=exp(-1j*pi*3/16)  OutDataTypeStr=const  SampleTime=-1
  Constant4 : Constant  Value=exp(-1j*pi*5/16)  OutDataTypeStr=const  SampleTime=-1
  Constant5 : Constant  Value=exp(-1j*pi*3/8)  OutDataTypeStr=const  SampleTime=-1
  Constant6 : Constant  Value=exp(-1j*pi*5/8)  OutDataTypeStr=const  SampleTime=-1
  Constant7 : Constant  Value=exp(-1j*pi*7/16)  OutDataTypeStr=const  SampleTime=-1
  Constant8 : Constant  Value=exp(-1j*pi*9/16)  OutDataTypeStr=const  SampleTime=-1
  Constant9 : Constant  Value=exp(-1j*pi*11/16)  OutDataTypeStr=const  SampleTime=-1
  Delay{,9..15,17,20..21,25,28..47} (32 alike) : Delay
  Delay{1..8,16,18..19,22..24,26..27,48,50..68,72,76} (38 alike) : Delay  DelayLength=3
  Delay{49,69..71,73..75,77..83} (14 alike) : Delay  DelayLength=1
  FFT16 : Subsystem
  FFT16_1 : Subsystem
  complexmult : Subsystem
  complexmult1 : Subsystem
  complexmult10 : Subsystem
  complexmult11 : Subsystem
  complexmult2 : Subsystem
  complexmult3 : Subsystem
  complexmult4 : Subsystem
  complexmult5 : Subsystem
  complexmult6 : Subsystem
  complexmult7 : Subsystem
  complexmult8 : Subsystem
  complexmult9 : Subsystem
  multByExp(-j*Pi/4) : Subsystem
  multByExp(-j*Pi/4)1 : Subsystem
  multByMinusJ : Subsystem
  multByMinusJ3 : Subsystem
  x0 : Outport  VectorParamsAs1DForOutWhenUnconnected=off
  x1 : Outport  Port=2  VectorParamsAs1DForOutWhenUnconnected=off
  x2 : Outport  Port=3  VectorParamsAs1DForOutWhenUnconnected=off
  x3 : Outport  Port=4  VectorParamsAs1DForOutWhenUnconnected=off
  x4 : Outport  Port=5  VectorParamsAs1DForOutWhenUnconnected=off
  x5 : Outport  Port=6  VectorParamsAs1DForOutWhenUnconnected=off
  x6 : Outport  Port=7  VectorParamsAs1DForOutWhenUnconnected=off
  x7 : Outport  Port=8  VectorParamsAs1DForOutWhenUnconnected=off
  x8 : Outport  Port=9  VectorParamsAs1DForOutWhenUnconnected=off
  x9 : Outport  Port=10  VectorParamsAs1DForOutWhenUnconnected=off
  x10 : Outport  Port=11  VectorParamsAs1DForOutWhenUnconnected=off
  x11 : Outport  Port=12  VectorParamsAs1DForOutWhenUnconnected=off
  x12 : Outport  Port=13  VectorParamsAs1DForOutWhenUnconnected=off
  x13 : Outport  Port=14  VectorParamsAs1DForOutWhenUnconnected=off
  x14 : Outport  Port=15  VectorParamsAs1DForOutWhenUnconnected=off
  x15 : Outport  Port=16  VectorParamsAs1DForOutWhenUnconnected=off
  x16 : Outport  Port=17  VectorParamsAs1DForOutWhenUnconnected=off
  x17 : Outport  Port=18  VectorParamsAs1DForOutWhenUnconnected=off
  x18 : Outport  Port=19  VectorParamsAs1DForOutWhenUnconnected=off
  x19 : Outport  Port=20  VectorParamsAs1DForOutWhenUnconnected=off
  x20 : Outport  Port=21  VectorParamsAs1DForOutWhenUnconnected=off
  x21 : Outport  Port=22  VectorParamsAs1DForOutWhenUnconnected=off
  x22 : Outport  Port=23  VectorParamsAs1DForOutWhenUnconnected=off
  x23 : Outport  Port=24  VectorParamsAs1DForOutWhenUnconnected=off
  x24 : Outport  Port=25  VectorParamsAs1DForOutWhenUnconnected=off
  x25 : Outport  Port=26  VectorParamsAs1DForOutWhenUnconnected=off
  x26 : Outport  Port=27  VectorParamsAs1DForOutWhenUnconnected=off
  x27 : Outport  Port=28  VectorParamsAs1DForOutWhenUnconnected=off
  x28 : Outport  Port=29  VectorParamsAs1DForOutWhenUnconnected=off
  x29 : Outport  Port=30  VectorParamsAs1DForOutWhenUnconnected=off
  x30 : Outport  Port=31  VectorParamsAs1DForOutWhenUnconnected=off
  x31 : Outport  Port=32  VectorParamsAs1DForOutWhenUnconnected=off
  wires:
  Delay83/1 -> Add23/2, Add22/2
  Delay82/1 -> Add21/2, Add20/2
  Delay81/1 -> Add19/2, Add18/2
  Delay80/1 -> multByMinusJ3/1(In1)
  Delay79/1 -> Add29/2, Add28/2
  Delay78/1 -> Add27/2, Add26/2
  Delay77/1 -> Add24/2, Add25/2
  Delay76/1 -> Add17/2, Add16/2
  Delay75/1 -> Add15/2, Add14/2
  Delay74/1 -> Add13/2, Add12/2
  Delay73/1 -> Add10/2, Add11/2
  Delay72/1 -> Add8/2, Add9/2
  Delay71/1 -> Add6/2, Add7/2
  Delay70/1 -> Add4/2, Add5/2
  Delay69/1 -> Add2/2, Add3/2
  Delay68/1 -> Add1/2, Add/2
  Delay67/1 -> Add23/1, Add22/1
  Delay66/1 -> Add20/1, Add21/1
  Delay65/1 -> Add19/1, Add18/1
  Delay64/1 -> Add30/1, Add31/1
  Delay52/1 -> Add29/1, Add28/1
  Delay62/1 -> Add27/1, Add26/1
  Delay56/1 -> Add25/1, Add24/1
  Delay63/1 -> Add17/1, Add16/1
  Delay61/1 -> Add14/1, Add15/1
  Delay60/1 -> Add13/1, Add12/1
  Delay59/1 -> Add10/1, Add11/1
  Delay58/1 -> Add9/1, Add8/1
  Delay53/1 -> Add6/1, Add7/1
  Delay55/1 -> Add4/1, Add5/1
  Delay54/1 -> Add2/1, Add3/1
  Delay57/1 -> Add1/1, Add/1
  Delay45/1 -> x30/1
  Delay43/1 -> x29/1
  Delay41/1 -> x28/1
  Delay39/1 -> x27/1
  Delay37/1 -> x26/1
  Delay35/1 -> x25/1
  Delay33/1 -> x24/1
  Delay31/1 -> x23/1
  Delay29/1 -> x22/1
  Delay25/1 -> x21/1
  Delay20/1 -> x20/1
  Delay15/1 -> x19/1
  Delay47/1 -> x31/1
  Delay21/1 -> x5/1
  Delay17/1 -> x4/1
  Delay13/1 -> x18/1
  Delay11/1 -> x17/1
  Delay9/1 -> x16/1
  Delay46/1 -> x15/1
  Delay44/1 -> x14/1
  Delay42/1 -> x13/1
  Delay40/1 -> x12/1
  Delay38/1 -> x11/1
  Delay36/1 -> x10/1
  Delay34/1 -> x9/1
  Delay28/1 -> x6/1
  Delay32/1 -> x8/1
  Delay30/1 -> x7/1
  Delay14/1 -> x3/1
  Delay12/1 -> x2/1
  Delay10/1 -> x1/1
  Delay/1 -> x0/1
  complexmult11/1(Out1) -> Delay83/1
  complexmult10/1(Out1) -> Delay82/1
  complexmult9/1(Out1) -> Delay81/1
  Delay51/1 -> Add31/2, Add30/2
  complexmult8/1(Out1) -> Delay79/1
  complexmult7/1(Out1) -> Delay78/1
  complexmult6/1(Out1) -> Delay77/1
  Delay50/1 -> Delay76/1
  complexmult5/1(Out1) -> Delay75/1
  complexmult4/1(Out1) -> Delay74/1
  complexmult3/1(Out1) -> Delay73/1
  Constant13/1 -> complexmult11/2(In3)
  Constant12/1 -> complexmult10/2(In3)
  FFT16_1/16(x15) -> complexmult11/1(x1)
  FFT16_1/15(x14) -> complexmult10/1(x1)
  FFT16_1/13(x12) -> multByExp(-j*Pi/4)1/1(x4)
  FFT16_1/14(x13) -> complexmult9/1(x1)
  Constant10/1 -> complexmult9/2(In3)
  Constant9/1 -> complexmult8/2(In3)
  FFT16_1/12(x11) -> complexmult8/1(x1)
  Constant6/1 -> complexmult7/2(In3)
  FFT16_1/11(x10) -> complexmult7/1(x1)
  Constant8/1 -> complexmult6/2(In3)
  FFT16_1/10(x9) -> complexmult6/1(x1)
  Constant7/1 -> complexmult5/2(In3)
  FFT16_1/8(x7) -> complexmult5/1(x1)
  Constant5/1 -> complexmult4/2(In3)
  FFT16_1/7(x6) -> complexmult4/1(x1)
  Constant4/1 -> complexmult3/2(In3)
  FFT16_1/6(x5) -> complexmult3/1(x1)
  multByMinusJ3/1(Out1) -> Delay51/1
  multByExp(-j*Pi/4)1/1(Out1) -> Delay80/1
  FFT16_1/9(x8) -> multByMinusJ/1(x4)
  multByMinusJ/1(Out1) -> Delay50/1
  Delay49/1 -> Delay72/1
  FFT16_1/5(x4) -> multByExp(-j*Pi/4)/1(x4)
  multByExp(-j*Pi/4)/1(Out1) -> Delay49/1
  complexmult2/1(Out1) -> Delay71/1
  Constant3/1 -> complexmult2/2(In3)
  FFT16_1/4(x3) -> complexmult2/1(x1)
  complexmult1/1(Out1) -> Delay70/1
  Constant1/1 -> complexmult1/2(In3)
  FFT16_1/3(x2) -> complexmult1/1(x1)
  complexmult/1(Out1) -> Delay69/1
  Constant2/1 -> complexmult/2(In3)
  FFT16_1/2(x1) -> complexmult/1(x1)
  Delay8/1 -> Delay67/1
  Delay7/1 -> Delay66/1
  Delay6/1 -> Delay65/1
  Delay5/1 -> Delay64/1
  Delay1/1 -> Delay52/1
  Delay3/1 -> Delay62/1
  Delay2/1 -> Delay56/1
  Delay4/1 -> Delay63/1
  Delay27/1 -> Delay61/1
  Delay26/1 -> Delay60/1
  Delay24/1 -> Delay59/1
  Delay23/1 -> Delay58/1
  Delay16/1 -> Delay53/1
  Delay19/1 -> Delay55/1
  Delay18/1 -> Delay54/1
  Delay48/1 -> Delay68/1
  FFT16_1/1(x0) -> Delay48/1
  Delay22/1 -> Delay57/1
  Add27/1 -> Delay37/1
  Add16/1 -> Delay32/1
  Add23/1 -> Delay47/1
  Add30/1 -> Delay40/1
  Add24/1 -> Delay34/1
  Add28/1 -> Delay38/1
  Add22/1 -> Delay46/1
  Add26/1 -> Delay36/1
  Add31/1 -> Delay41/1
  Add17/1 -> Delay33/1
  Add29/1 -> Delay39/1
  Add19/1 -> Delay43/1
  Add25/1 -> Delay35/1
  Add21/1 -> Delay45/1
  Add20/1 -> Delay44/1
  Add18/1 -> Delay42/1
  Add2/1 -> Delay10/1
  Add9/1 -> Delay20/1
  Add8/1 -> Delay17/1
  Add14/1 -> Delay30/1
  Add12/1 -> Delay28/1
  Add15/1 -> Delay31/1
  Add3/1 -> Delay11/1
  Add4/1 -> Delay12/1
  Add10/1 -> Delay21/1
  Add/1 -> Delay/1
  Add5/1 -> Delay13/1
  Add13/1 -> Delay29/1
  Add6/1 -> Delay14/1
  Add11/1 -> Delay25/1
  Add7/1 -> Delay15/1
  Add1/1 -> Delay9/1
  FFT16/16(x15) -> Delay8/1
  FFT16/9(x8) -> Delay4/1
  FFT16/15(x14) -> Delay7/1
  FFT16/10(x9) -> Delay2/1
  FFT16/14(x13) -> Delay6/1
  FFT16/11(x10) -> Delay3/1
  FFT16/13(x12) -> Delay5/1
  FFT16/12(x11) -> Delay1/1
  FFT16/8(x7) -> Delay27/1
  FFT16/7(x6) -> Delay26/1
  FFT16/6(x5) -> Delay24/1
  FFT16/5(x4) -> Delay23/1
  FFT16/4(x3) -> Delay16/1
  FFT16/3(x2) -> Delay19/1
  FFT16/2(x1) -> Delay18/1
  FFT16/1(x0) -> Delay22/1
  In32/1 -> FFT16_1/16(In16)
  In30/1 -> FFT16_1/15(In15)
  In28/1 -> FFT16_1/14(In14)
  In26/1 -> FFT16_1/13(In13)
  In24/1 -> FFT16_1/12(In12)
  In22/1 -> FFT16_1/11(In11)
  In20/1 -> FFT16_1/10(In10)
  In16/1 -> FFT16_1/9(In9)
  In17/1 -> FFT16_1/8(In8)
  In14/1 -> FFT16_1/7(In7)
  In12/1 -> FFT16_1/6(In6)
  In10/1 -> FFT16_1/5(In5)
  In8/1 -> FFT16_1/4(In4)
  In6/1 -> FFT16_1/3(In3)
  In4/1 -> FFT16_1/2(In2)
  In2/1 -> FFT16_1/1(In1)
  In31/1 -> FFT16/16(In16)
  In29/1 -> FFT16/15(In15)
  In27/1 -> FFT16/14(In14)
  In25/1 -> FFT16/13(In13)
  In23/1 -> FFT16/12(In12)
  In21/1 -> FFT16/11(In11)
  In18/1 -> FFT16/10(In10)
  In19/1 -> FFT16/9(In9)
  In15/1 -> FFT16/8(In8)
  In13/1 -> FFT16/7(In7)
  In11/1 -> FFT16/6(In6)
  In9/1 -> FFT16/5(In5)
  In7/1 -> FFT16/4(In4)
  In5/1 -> FFT16/3(In3)
  In3/1 -> FFT16/2(In2)
  In1/1 -> FFT16/1(In1)
